simulink model "system2_time"  (R2019b)
settings: Solver=VariableStepAuto  StartTime=0.0  StopTime=10.0  RelTol=1e-3
settings Model: Creator=davis  LastModifiedBy=davis

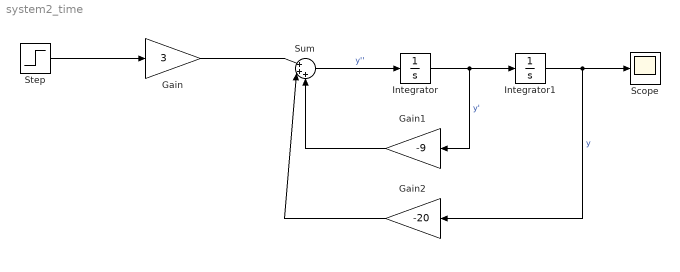
== system system2_time ==
  Gain : Gain  Gain=3
  Gain1 : Gain  Gain=-9
  Gain2 : Gain  Gain=-20
  Integrator : Integrator  InitialCondition=2
  Integrator1 : Integrator  InitialCondition=3
  Scope : Scope
  Step : Step  Time=0  SampleTime=0
  Sum : Sum  Inputs=|+++
  wires:
  Sum/1 -> Integrator/1  "y''"
  Integrator/1 -> Gain1/1, Integrator1/1  "y'"
  Gain1/1 -> Sum/3
  Gain2/1 -> Sum/2
  Gain/1 -> Sum/1
  Integrator1/1 -> Gain2/1, Scope/1  "y"
  Step/1 -> Gain/1
